simulink model "ComboStickmanARev2022a"  (R2022a)
settings: Solver=VariableStepAuto  StartTime=0.0  StopTime=18  RelTol=1e-3
libraries: aerolibanim x1, shared6dof x1
settings Model: PacingRate=0.500000  Creator=mthorbu  LastModifiedBy=mthorbu

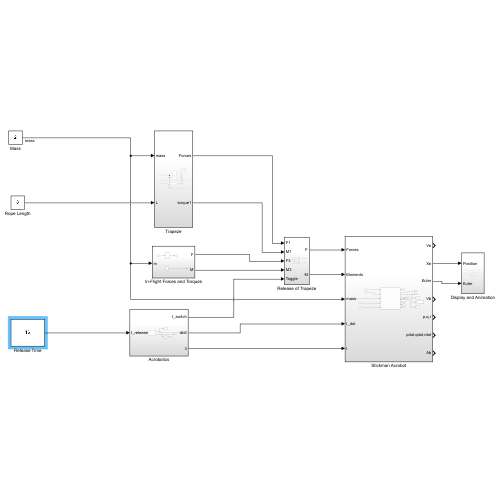
[thumbnail: Simulink's stored preview of the top-level diagram]
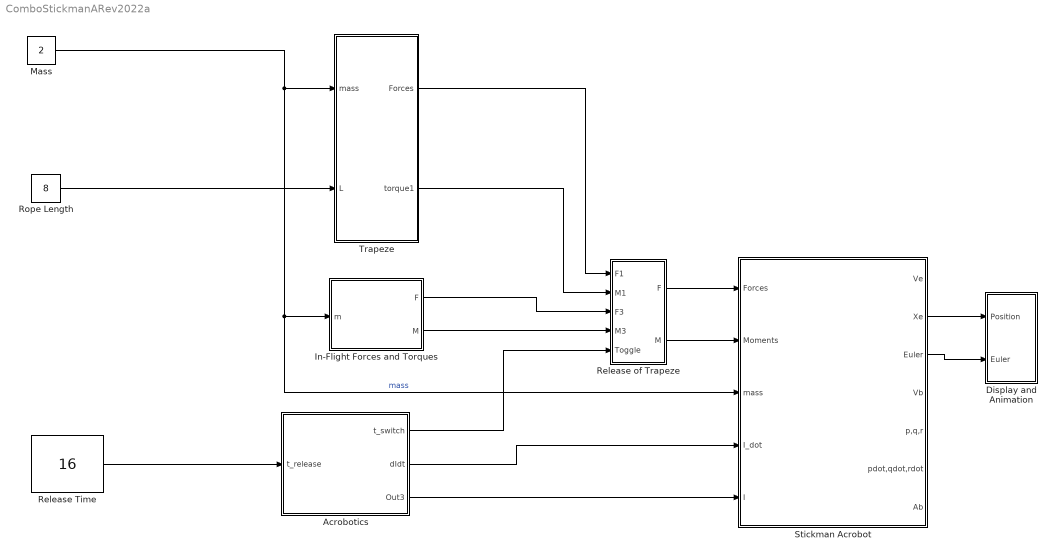
== system ComboStickmanARev2022a ==
  Acrobotics : Subsystem
  Display and Animation : Subsystem
  In-Flight Forces and Torques : Subsystem
  Mass : Constant  Value=2
  Release Time : Constant  Value=16
  Release of Trapeze : Subsystem
  Rope Length : Constant  Value=8
  Stickman Acrobot : Subsystem
  Trapeze : Subsystem
  wires:
  Stickman Acrobot/2(Xe) -> Display and Animation/1(Position)
  Stickman Acrobot/3(Euler) -> Display and Animation/2(Euler)
  Mass/1 -> Stickman Acrobot/3(mass), In-Flight Forces and Torques/1(m), Trapeze/1(mass)  "mass"
  Rope Length/1 -> Trapeze/2(L)
  Release Time/1 -> Acrobotics/1(t_release)
  Acrobotics/2(dIdt) -> Stickman Acrobot/4(I_dot)
  Acrobotics/3(Out3) -> Stickman Acrobot/5(I)
  Trapeze/1(Forces) -> Release of Trapeze/1(F1)
  Trapeze/2(torque1) -> Release of Trapeze/2(M1)
  In-Flight Forces and Torques/1(F) -> Release of Trapeze/3(F3)
  Acrobotics/1(t_switch) -> Release of Trapeze/5(Toggle)
  In-Flight Forces and Torques/2(M) -> Release of Trapeze/4(M3)
  Release of Trapeze/1(F) -> Stickman Acrobot/1(Forces)
  Release of Trapeze/2(M) -> Stickman Acrobot/2(Moments)

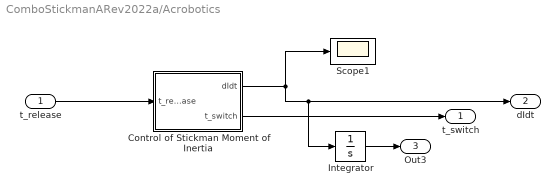
== system ComboStickmanARev2022a/Acrobotics ==
  t_release : Inport
  Control of Stickman Moment of Inertia : Stateflow chart  TreatAsAtomicUnit=on
  Integrator : Integrator  InitialCondition=eye(3)
  Scope1 : Scope
  t_switch : Outport
  dIdt : Outport  Port=2
  Out3 : Outport  Port=3
  wires:
  Control of Stickman Moment of Inertia/1(dIdt) -> dIdt/1, Integrator/1, Scope1/1
  t_release/1 -> Control of Stickman Moment of Inertia/1(t_release)
  Integrator/1 -> Out3/1
  Control of Stickman Moment of Inertia/2(t_switch) -> t_switch/1

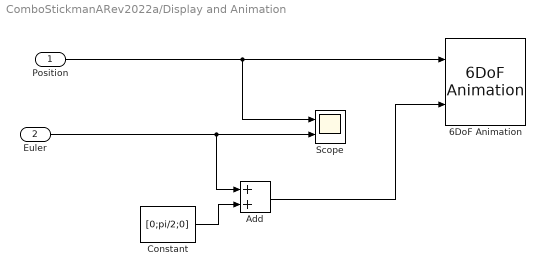
== system ComboStickmanARev2022a/Display and Animation ==
  Position : Inport
  Euler : Inport  Port=2
  6DoF Animation : aerolibanim/6DoF Animation  u1=[-50 50 -50 50 -100 0]  u2=0.05  u3=3.0  u4=[0,0,0]  u5=Fixed position  u6=[10,10,0]  u7=90  u8=on
  Add : Sum
  Constant : Constant  Value=[0;pi/2;0]
  Scope : Scope  NumInputPorts=2
  wires:
  Euler/1 -> Scope/2, Add/1
  Position/1 -> Scope/1, 6DoF Animation/1
  Constant/1 -> Add/2
  Add/1 -> 6DoF Animation/2

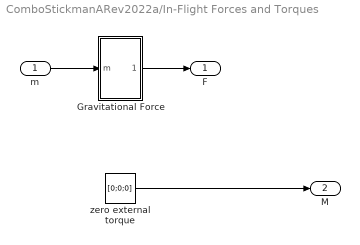
== system ComboStickmanARev2022a/In-Flight Forces and Torques ==
  m : Inport
  Gravitational Force : Subsystem
  zero external torque : Constant  Value=[0;0;0]
  F : Outport
  M : Outport  Port=2
  wires:
  zero external torque/1 -> M/1
  m/1 -> Gravitational Force/1(m)
  Gravitational Force/1(Out1) -> F/1

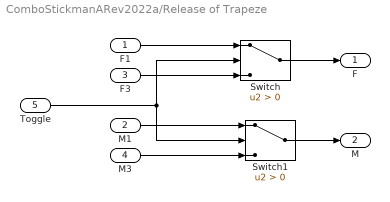
== system ComboStickmanARev2022a/Release of Trapeze ==
  F1 : Inport
  M1 : Inport  Port=2
  F3 : Inport  Port=3
  M3 : Inport  Port=4
  Toggle : Inport  Port=5
  Switch : Switch  Criteria=u2 > Threshold  SaturateOnIntegerOverflow=off  InputSameDT=off
  Switch1 : Switch  Criteria=u2 > Threshold  SaturateOnIntegerOverflow=off  InputSameDT=off
  F : Outport
  M : Outport  Port=2
  wires:
  M1/1 -> Switch1/1
  Switch/1 -> F/1
  M3/1 -> Switch1/3
  Switch1/1 -> M/1
  Toggle/1 -> Switch1/2, Switch/2
  F1/1 -> Switch/1
  F3/1 -> Switch/3

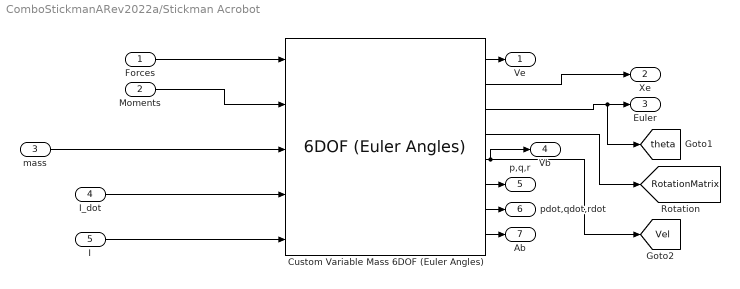
== system ComboStickmanARev2022a/Stickman Acrobot ==
  Forces : Inport
  Moments : Inport  Port=2
  mass : Inport  Port=3
  I_dot : Inport  Port=4
  I : Inport  Port=5
  Custom Variable Mass 6DOF (Euler Angles) : shared6dof/6DOF (Euler Angles)  units=Metric (MKS)  mtype=Custom Variable  rep=Euler Angles  xme_0=[-8 0 -8]  Vm_0=[0 0 0]  eul_0=[0 -pi/2 0]  pm_0=[0 0 0]  mass_0=1.0  mass_e=0.5  mass_f=2.0  inertia=eye(3)  inertia_e=eye(3)  inertia_f=2*eye(3)  k_quat=1.0  vre_flag=off  abi_flag=off  aMode=0  xme_statename=''  Vm_statename=''  eul_statename=''  quat_statename=''  pm_statename=''  mass_statename=''
      settings: SourceProductBaseCode=AE,PW,DR,MT,VE
  Ve : Outport
  Xe : Outport  Port=2
  Euler : Outport  Port=3
  Vb : Outport  Port=4
  p,q,r : Outport  Port=5
  pdot,qdot,rdot : Outport  Port=6
  Ab : Outport  Port=7
  tag scope: RotationMatrix=global, Vel=global, theta=global
  wires:
  Custom Variable Mass 6DOF (Euler Angles)/6 -> p,q,r/1
  Moments/1 -> Custom Variable Mass 6DOF (Euler Angles)/2
  Custom Variable Mass 6DOF (Euler Angles)/1 -> Ve/1
  Custom Variable Mass 6DOF (Euler Angles)/4 -> [RotationMatrix]
  Forces/1 -> Custom Variable Mass 6DOF (Euler Angles)/1
  Custom Variable Mass 6DOF (Euler Angles)/3 -> [theta], Euler/1
  I_dot/1 -> Custom Variable Mass 6DOF (Euler Angles)/4
  Custom Variable Mass 6DOF (Euler Angles)/2 -> Xe/1
  Custom Variable Mass 6DOF (Euler Angles)/5 -> [Vel], Vb/1
  I/1 -> Custom Variable Mass 6DOF (Euler Angles)/5
  Custom Variable Mass 6DOF (Euler Angles)/7 -> pdot,qdot,rdot/1
  Custom Variable Mass 6DOF (Euler Angles)/8 -> Ab/1
  mass/1 -> Custom Variable Mass 6DOF (Euler Angles)/3

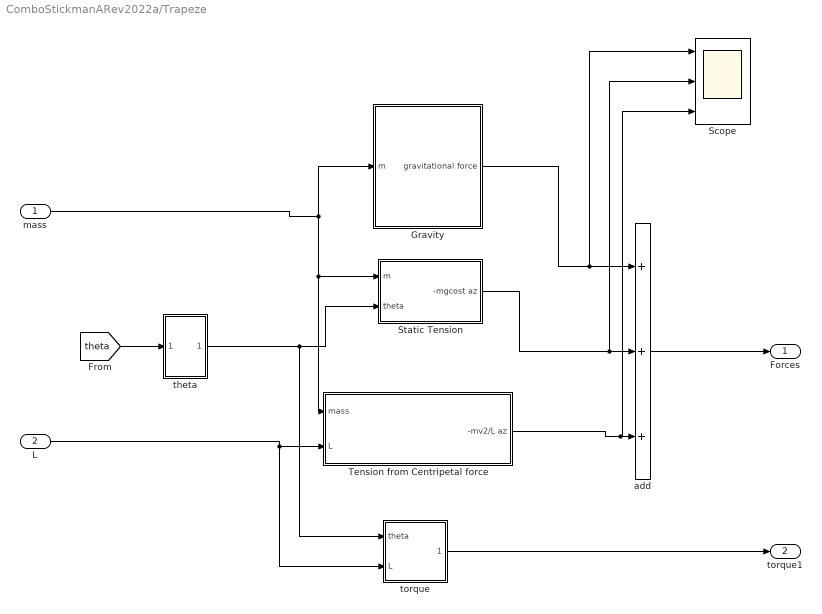
== system ComboStickmanARev2022a/Trapeze ==
  mass : Inport
  L : Inport  Port=2
  Gravity : Subsystem
  Scope : Scope  NumInputPorts=3
  Static Tension : Subsystem
  Tension from Centripetal force : Subsystem
  add : Sum  Inputs=+++
  theta : Subsystem
  torque : Subsystem
  Forces : Outport
  torque1 : Outport  Port=2
  wires:
  theta/1(Out1) -> torque/1(theta), Static Tension/2(theta)
  [theta] -> theta/1(In1)
  mass/1 -> Tension from Centripetal force/1(mass), Static Tension/1(m), Gravity/1(m)
  Tension from Centripetal force/1(-mv2/L az) -> Scope/3, add/3
  Static Tension/1(-mgcost az) -> Scope/2, add/2
  Gravity/1(gravitational force) -> Scope/1, add/1
  L/1 -> torque/2(L), Tension from Centripetal force/2(L)
  add/1 -> Forces/1
  torque/1(torque) -> torque1/1

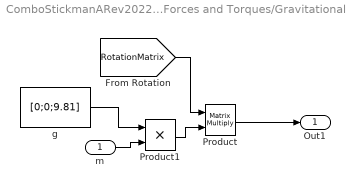
== system ComboStickmanARev2022a/In-Flight Forces and Torques/Gravitational Force ==
  m : Inport
  Product : Product  Multiplication=Matrix(*)
  Product1 : Product
  g : Constant  Value=[0;0;9.81]
  Out1 : Outport
  wires:
  [RotationMatrix] -> Product/1
  g/1 -> Product1/1
  Product1/1 -> Product/2
  Product/1 -> Out1/1
  m/1 -> Product1/2

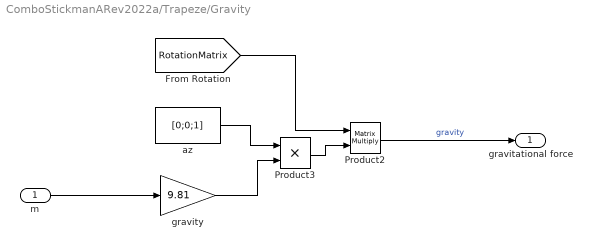
== system ComboStickmanARev2022a/Trapeze/Gravity ==
  m : Inport
  Product2 : Product  Multiplication=Matrix(*)
  Product3 : Product
  az : Constant  Value=[0;0;1]
  gravity : Gain  Gain=9.81
  gravitational force : Outport
  wires:
  [RotationMatrix] -> Product2/1
  az/1 -> Product3/1
  gravity/1 -> Product3/2
  Product3/1 -> Product2/2
  Product2/1 -> gravitational force/1  "gravity"
  m/1 -> gravity/1

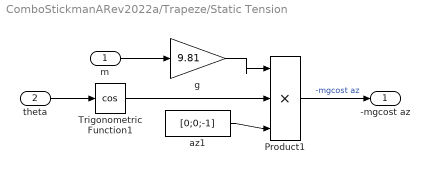
== system ComboStickmanARev2022a/Trapeze/Static Tension ==
  m : Inport
  theta : Inport  Port=2
  Product1 : Product  Inputs=3
  Trigonometric Function1 : Trigonometry  Operator=cos
  az1 : Constant  Value=[0;0;-1]
  g : Gain  Gain=9.81
  -mgcost az : Outport
  wires:
  m/1 -> g/1
  az1/1 -> Product1/3
  Trigonometric Function1/1 -> Product1/2
  g/1 -> Product1/1
  theta/1 -> Trigonometric Function1/1
  Product1/1 -> -mgcost az/1  "-mgcost az"

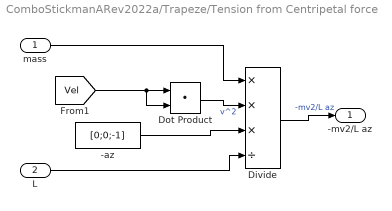
== system ComboStickmanARev2022a/Trapeze/Tension from Centripetal force ==
  mass : Inport
  L : Inport  Port=2
  -az : Constant  Value=[0;0;-1]
  Divide : Product  Inputs=***/
  Dot Product : DotProduct  OutDataTypeStr=Inherit: Inherit via internal rule
  -mv2/L az : Outport
  wires:
  -az/1 -> Divide/3
  [Vel] -> Dot Product/2, Dot Product/1
  Dot Product/1 -> Divide/2  "v^2"
  L/1 -> Divide/4
  Divide/1 -> -mv2/L az/1  "-mv2/L az"
  mass/1 -> Divide/1

== system ComboStickmanARev2022a/Trapeze/theta ==
  In1 : Inport
  Demux : Demux  Outputs=3
  Terminator : Terminator
  Terminator1 : Terminator
  Out1 : Outport
  wires:
  Demux/3 -> Terminator1/1
  Demux/1 -> Terminator/1
  Demux/2 -> Out1/1
  In1/1 -> Demux/1

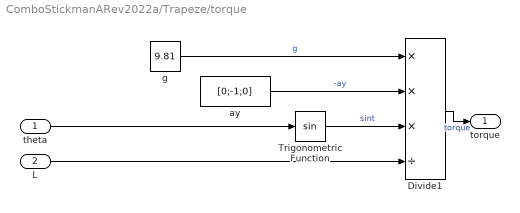
== system ComboStickmanARev2022a/Trapeze/torque ==
  theta : Inport
  L : Inport  Port=2
  Divide1 : Product  Inputs=***/
  Trigonometric Function : Trigonometry
  ay : Constant  Value=[0;-1;0]
  g : Constant  Value=9.81
  torque : Outport
  wires:
  theta/1 -> Trigonometric Function/1
  L/1 -> Divide1/4
  g/1 -> Divide1/1  "g"
  ay/1 -> Divide1/2  "-ay"
  Trigonometric Function/1 -> Divide1/3  "sint"
  Divide1/1 -> torque/1  "torque"

== stateflow chart ComboStickmanARev2022a/Acrobotics/Control of Stickman Moment of Inertia ==
  state Initialize
    entry:
    t_switch=1;
    dIdt=0*eye(3);
  state Release
    entry:
    t_switch=0;
    dIdt=0*eye(3);
  state transiton
    entry:
    dIdt=-8*eye(3);
  state transiton2
    entry:
    dIdt=0*eye(3);
  (default) -> Initialize
  Initialize -> Release : [after(t_release,sec)]
  Release -> transiton : [after(0.2,sec)]
  transiton -> transiton2 : [after(0.1,sec)]
  data: dIdt output; t_release input; t_switch output
